simulink model "FSK_3"  (R2017b)
settings: Solver=VariableStepAuto  StartTime=0.0  StopTime=10  MaxStep=0.01  MinStep=0.001  RelTol=1e-3
libraries: dsparch4 x5, neural x2, commchan3 x1
settings Model: Creator=ayadd  LastModifiedBy=ayadd
settings SolverCC: ShapePreserveControl=EnableAll  ZeroCrossAlgorithm=Adaptive

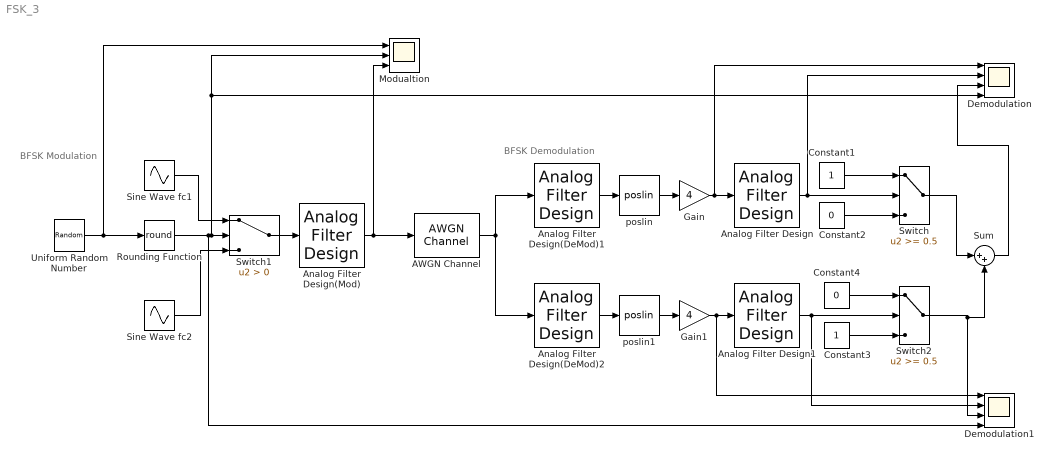
== system FSK_3 ==
  note: BFSK Demodulation
  note: BFSK Modulation
  AWGN Channel : commchan3/AWGN Channel  InputProcessing=Columns as channels (frame based)  seed=67  noiseMode="Signal to noise ratio  (SNR)"  EbNodB=10  EsNodB=10  SNRdB=70  bitsPerSym=1  Ps=1  Tsym=1  variance=1
  Analog Filter Design : dsparch4/Analog Filter Design  method=Butterworth  filttype=Lowpass  N=8  Wlo=30  Whi=80  Rp=2  Rs=40
  Analog Filter Design(DeMod)1 : dsparch4/Analog Filter Design  method=Butterworth  filttype=Bandpass  N=10  Wlo=10*2*pi  Whi=20*2*pi  Rp=2  Rs=40
  Analog Filter Design(DeMod)2 : dsparch4/Analog Filter Design  method=Butterworth  filttype=Bandpass  N=10  Wlo=0.16  Whi=8*2*pi  Rp=2  Rs=40
  Analog Filter Design(Mod) : dsparch4/Analog Filter Design  method=Butterworth  filttype=Bandpass  N=10  Wlo=0.16  Whi=350  Rp=2  Rs=40
  Analog Filter Design1 : dsparch4/Analog Filter Design  method=Butterworth  filttype=Lowpass  N=8  Wlo=20  Whi=80  Rp=2  Rs=40
  Constant1 : Constant
  Constant2 : Constant  Value=0
  Constant3 : Constant
  Constant4 : Constant  Value=0
  Demodulation : Scope  NumInputPorts=4
  Demodulation1 : Scope  NumInputPorts=4
  Gain : Gain  Gain=4
  Gain1 : Gain  Gain=4
  Modualtion : Scope  NumInputPorts=3
  Rounding Function : Rounding  Operator=round
  Sine Wave fc1 : Sin  Frequency=15*2*pi  SampleTime=0
  Sine Wave fc2 : Sin  Frequency=5*2*pi  SampleTime=0
  Sum : Sum  Inputs=|++
  Switch : Switch  Threshold=0.5  RndMeth=Round  SaturateOnIntegerOverflow=on  InputSameDT=on
  Switch1 : Switch  Criteria=u2 > Threshold
  Switch2 : Switch  Threshold=0.5  RndMeth=Round  SaturateOnIntegerOverflow=on  InputSameDT=on
  Uniform Random Number : UniformRandomNumber  Minimum=0  SampleTime=1
  poslin : neural/Transfer Functions/poslin
      settings: SourceProductName=Neural Network Toolbox  SourceProductBaseCode=NN
  poslin1 : neural/Transfer Functions/poslin
      settings: SourceProductName=Neural Network Toolbox  SourceProductBaseCode=NN
  wires:
  Analog Filter Design/1 -> Demodulation/2, Switch/2
  Gain/1 -> Demodulation/1, Analog Filter Design/1
  Switch/1 -> Sum/1
  Constant1/1 -> Switch/1
  Constant2/1 -> Switch/3
  poslin/1 -> Gain/1
  Switch1/1 -> Analog Filter Design(Mod)/1
  Sine Wave fc1/1 -> Switch1/1
  Sine Wave fc2/1 -> Switch1/3
  Uniform Random Number/1 -> Modualtion/1, Rounding Function/1
  Rounding Function/1 -> Demodulation1/4, Modualtion/2, Demodulation/4, Switch1/2
  Analog Filter Design(Mod)/1 -> AWGN Channel/1, Modualtion/3
  AWGN Channel/1 -> Analog Filter Design(DeMod)1/1, Analog Filter Design(DeMod)2/1
  Analog Filter Design(DeMod)1/1 -> poslin/1
  poslin1/1 -> Gain1/1
  Gain1/1 -> Demodulation1/1, Analog Filter Design1/1
  Analog Filter Design(DeMod)2/1 -> poslin1/1
  Analog Filter Design1/1 -> Demodulation1/2, Switch2/2
  Constant4/1 -> Switch2/1
  Constant3/1 -> Switch2/3
  Switch2/1 -> Sum/2, Demodulation1/3
  Sum/1 -> Demodulation/3
